simulink model "svpwm3level"  (Simulink 7.1)
settings: Solver=ode3  StartTime=0.0  StopTime=1  RelTol=1e-3
libraries: powerlib x13, simulink x1
(part 1 of 2)
settings Model: Creator=ki  LastModifiedBy=Leavy

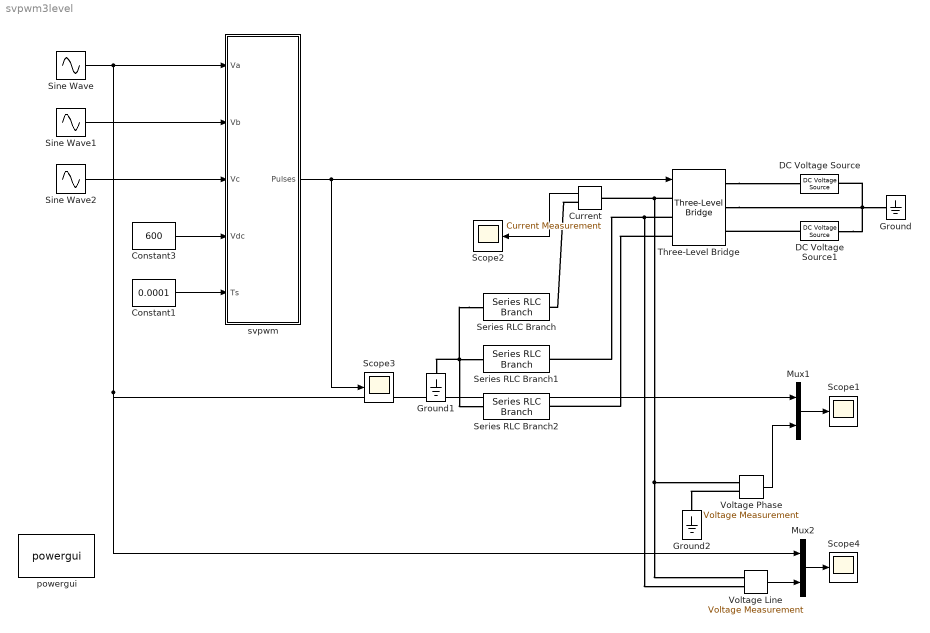
== system svpwm3level ==
  Constant1 : Constant  Value=0.0001  OutDataType=sfix(16)  OutScaling=2^0
  Constant3 : Constant  Value=600  OutDataType=sfix(16)  OutScaling=2^0
  "Current " : powerlib/Measurements/Current Measurement  Orientation=left  DialogController=POWERSYS.PowerSysDialog  SystemSampleTime=-1  PhasorSimulation=off  OutputType=Complex  PSBequivalent=0
  DC Voltage Source : powerlib/Electrical Sources/DC Voltage Source  Orientation=left  DialogController=POWERSYS.PowerSysDialog  SystemSampleTime=-1  Amplitude=300  Measurements=None
  DC Voltage Source1 : powerlib/Electrical Sources/DC Voltage Source  DialogController=POWERSYS.PowerSysDialog  SystemSampleTime=-1  Amplitude=300  Measurements=None
  Ground : powerlib/Elements/Ground  DialogController=POWERSYS.PowerSysDialog  PhysicalDomain=powersysdomain  SubClassName=unknown  LeftPortType=p1  RightPortType=p1  LConnTagsString=a
  Ground1 : powerlib/Elements/Ground  Orientation=down  DialogController=POWERSYS.PowerSysDialog  PhysicalDomain=powersysdomain  SubClassName=unknown  LeftPortType=p1  RightPortType=p1  LConnTagsString=a
  Ground2 : powerlib/Elements/Ground  Orientation=down  DialogController=POWERSYS.PowerSysDialog  PhysicalDomain=powersysdomain  SubClassName=unknown  LeftPortType=p1  RightPortType=p1  LConnTagsString=a
  Mux1 : Mux  Inputs=2
  Mux2 : Mux  Inputs=2
  Scope{1..4} (4 alike) : Scope
      Scope1 settings: TimeRange=0.01703035274815434  YMin=-350  YMax=350  MaxDataPoints=20000
      Scope2 settings: TimeRange=0.01703035274815434  YMin=-800  YMax=1500  SaveName=ScopeData2  MaxDataPoints=20000
      Scope3 settings: TimeRange=0.01703035274815434  YMin=-150  YMax=80  SaveName=ScopeData4  MaxDataPoints=20000
      Scope4 settings: TimeRange=0.01703035274815434  YMin=-700  YMax=700  SaveName=ScopeData15  MaxDataPoints=20000
  Series RLC Branch : powerlib/Elements/Series RLC Branch  DialogController=POWERSYS.PowerSysDialog  PhysicalDomain=powersysdomain  SubClassName=unknown  LeftPortType=p1  RightPortType=p1  LConnTagsString=__new0  RConnTagsString=__new0  BranchType=L  Resistance=10  Inductance=5e-4  SetiL0=off  InitialCurrent=0  Capacitance=1.0  Setx0=off  InitialVoltage=0  Measurements=None
  Series RLC Branch1 : powerlib/Elements/Series RLC Branch  DialogController=POWERSYS.PowerSysDialog  PhysicalDomain=powersysdomain  SubClassName=unknown  LeftPortType=p1  RightPortType=p1  LConnTagsString=__new0  RConnTagsString=__new0  BranchType=L  Resistance=10  Inductance=5e-4  SetiL0=off  InitialCurrent=0  Capacitance=1e-6  Setx0=off  InitialVoltage=0  Measurements=None
  Series RLC Branch2 : powerlib/Elements/Series RLC Branch  DialogController=POWERSYS.PowerSysDialog  PhysicalDomain=powersysdomain  SubClassName=unknown  LeftPortType=p1  RightPortType=p1  LConnTagsString=__new0  RConnTagsString=__new0  BranchType=L  Resistance=10  Inductance=5e-4  SetiL0=off  InitialCurrent=0  Capacitance=1e-6  Setx0=off  InitialVoltage=0  Measurements=None
  Sine Wave : Sin  Amplitude=220  Frequency=314  SampleTime=0
  Sine Wave1 : Sin  Amplitude=220  Frequency=314  Phase=-2*pi/3  SampleTime=0
  Sine Wave2 : Sin  Amplitude=220  Frequency=314  Phase=-4*pi/3  SampleTime=0
  Three-Level Bridge : powerlib/Power Electronics/Three-Level Bridge  DialogController=POWERSYS.PowerSysDialog  SystemSampleTime=-1  Arms=3  SnubberResistance=1e5  SbubberCapacitance=inf  Device=IGBT / Diodes  Ron=1e-3  ForwardVoltages="[  0  0  ]"  Measurements=None
  Voltage Line : powerlib/Measurements/Voltage Measurement  DialogController=POWERSYS.PowerSysDialog  SystemSampleTime=-1  PhasorSimulation=off  OutputType=Complex  PSBequivalent=0
  Voltage Phase : powerlib/Measurements/Voltage Measurement  DialogController=POWERSYS.PowerSysDialog  SystemSampleTime=-1  PhasorSimulation=off  OutputType=Complex  PSBequivalent=0
  powergui : powerlib/powergui  Priority=2  SystemSampleTime=-1  SimulationMode=Discrete  SampleTime=0.000002  frequency=60  SPID=off  SwTol=0  Interpol=off  x0status=blocks  echomessages=off  HookPort=off  FunctionMessages=off  EnableUseOfTLC=off  RestoreLinks=warning  frequencyindice=0  Frange=[0:2:500]  Ylog=off  Xlog=on  ShowGrid=off  save=off  variable=ZData  ZoomFFT=on  StartTime=0.0  cycles=1  DisplayStyle=1  fundamental=60  FreqAxis=off  MaxFrequency=1000  frequencyindicesteady=1  RmsSteady=1  display=off  Ts=0  methode=off
  svpwm : Subsystem
  wires:
  Constant3/1 -> svpwm/4(Vdc)
  Constant1/1 -> svpwm/5(Ts)
  svpwm/1(Pulses) -> Three-Level Bridge/1, Scope3/1
  Sine Wave2/1 -> svpwm/3(Vc)
  Sine Wave1/1 -> svpwm/2(Vb)
  Sine Wave/1 -> svpwm/1(Va), Mux1/1, Mux2/1
  "Current "/1 -> Scope2/1
  Voltage Phase/1 -> Mux1/2
  Mux1/1 -> Scope1/1
  Mux2/1 -> Scope4/1
  Voltage Line/1 -> Mux2/2
  connections:
  Three-Level Bridge/RConn1 -- DC Voltage Source/RConn1
  DC Voltage Source1/RConn1 -- DC Voltage Source/LConn1 -- Three-Level Bridge/RConn2 -- Ground/LConn1
  DC Voltage Source1/LConn1 -- Three-Level Bridge/RConn3
  Series RLC Branch/LConn1 -- Series RLC Branch1/LConn1 -- Series RLC Branch2/LConn1 -- Ground1/LConn1
  Three-Level Bridge/LConn2 -- Series RLC Branch1/RConn1 -- Voltage Line/LConn2
  Three-Level Bridge/LConn3 -- Series RLC Branch2/RConn1
  Three-Level Bridge/LConn1 -- "Current "/LConn1 -- Voltage Phase/LConn1 -- Voltage Line/LConn1
  "Current "/RConn1 -- Series RLC Branch/RConn1
  Voltage Phase/LConn2 -- Ground2/LConn1

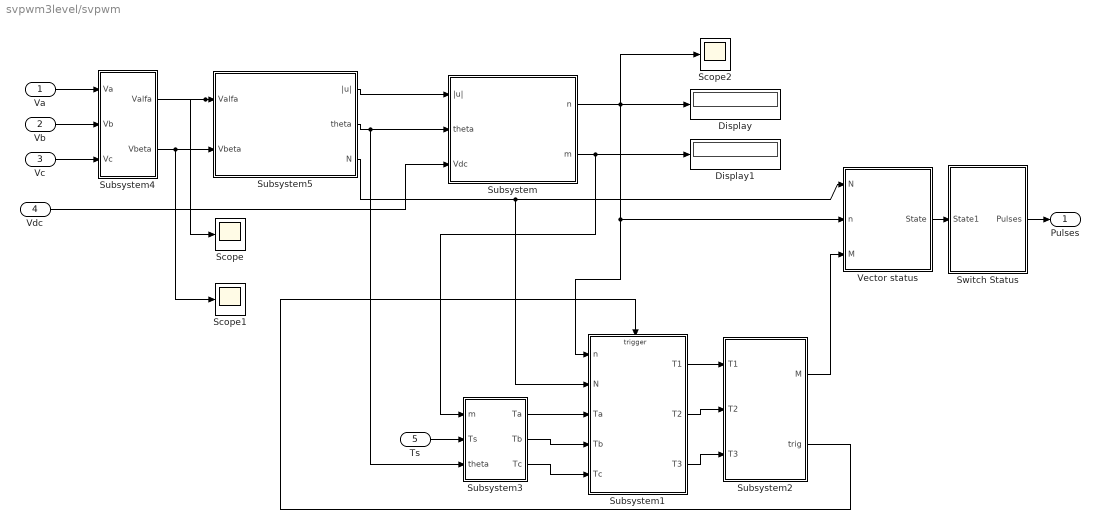
== system svpwm3level/svpwm ==
  Va : Inport  OutDataType=sfix(16)  OutScaling=2^0
  Vb : Inport  Port=2  OutDataType=sfix(16)  OutScaling=2^0
  Vc : Inport  Port=3  OutDataType=sfix(16)  OutScaling=2^0
  Vdc : Inport  Port=4  OutDataType=sfix(16)  OutScaling=2^0
  Ts : Inport  Port=5  OutDataType=sfix(16)  OutScaling=2^0
  Display : Display
  Display1 : Display
  Scope : Scope
      settings: YMin=-150  YMax=-150  SaveName=ScopeData6
  Scope1 : Scope
      settings: YMin=-606.218  YMax=-606.218  SaveName=ScopeData7
  Scope2 : Scope
      settings: YMin=3  YMax=6  SaveName=ScopeData8  MaxDataPoints=20000
  Subsystem : Subsystem
  Subsystem1 : Subsystem
  Subsystem2 : Subsystem
  Subsystem3 : Subsystem
  Subsystem4 : Subsystem
  Subsystem5 : Subsystem
  Switch Status : Subsystem
  Vector status : Subsystem
  Pulses : Outport  OutDataType=sfix(16)  OutScaling=2^0
  wires:
  Vc/1 -> Subsystem4/3(Vc)
  Subsystem4/2(Vbeta) -> Scope1/1, Subsystem5/2(Vbeta)
  Subsystem4/1(Valfa) -> Subsystem5/1(Valfa), Scope/1
  Vb/1 -> Subsystem4/2(Vb)
  Va/1 -> Subsystem4/1(Va)
  Vdc/1 -> Subsystem/3(Vdc)
  Ts/1 -> Subsystem3/2(Ts)
  Subsystem2/1(M) -> Vector status/3(M)
  Subsystem/2(m) -> Subsystem3/1(m), Display1/1
  Subsystem/1(n) -> Display/1, Scope2/1, Vector status/2(n), Subsystem1/1(n)
  Subsystem5/3(N) -> Vector status/1(N), Subsystem1/2(N)
  Subsystem5/1(|u|) -> Subsystem/1(|u|)
  Switch Status/1(Pulses) -> Pulses/1
  Vector status/1(State) -> Switch Status/1(State1)
  Subsystem5/2(theta) -> Subsystem/2(theta), Subsystem3/3(theta)
  Subsystem2/2(trig) -> Subsystem1/Trigger
  Subsystem3/1(Ta) -> Subsystem1/3(Ta)
  Subsystem3/2(Tb) -> Subsystem1/4(Tb)
  Subsystem3/3(Tc) -> Subsystem1/5(Tc)
  Subsystem1/1(T1) -> Subsystem2/1(T1)
  Subsystem1/2(T2) -> Subsystem2/2(T2)
  Subsystem1/3(T3) -> Subsystem2/3(T3)

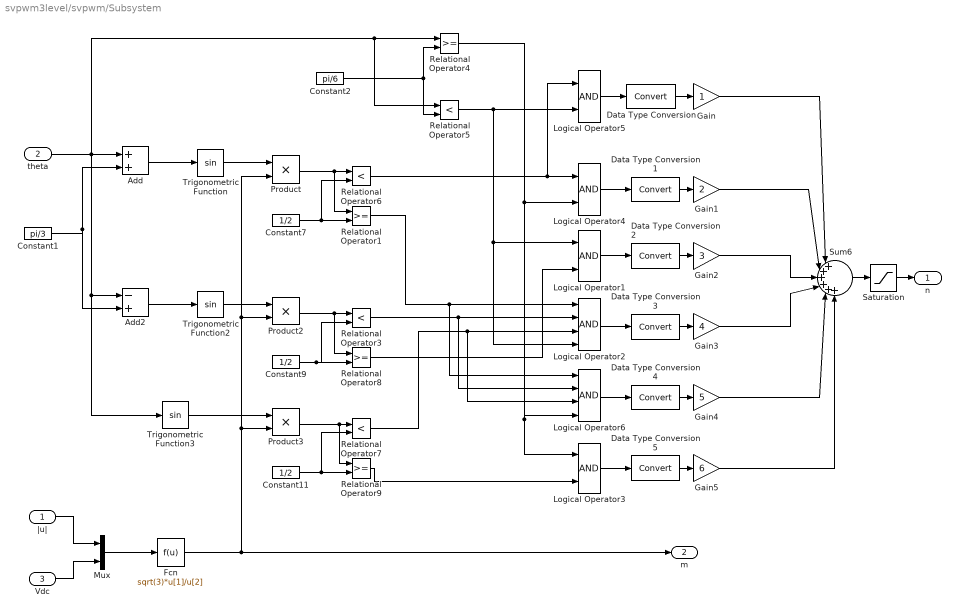
== system svpwm3level/svpwm/Subsystem ==
  |u| : Inport  OutDataType=sfix(16)  OutScaling=2^0
  theta : Inport  Port=2  OutDataType=sfix(16)  OutScaling=2^0
  Vdc : Inport  Port=3  OutDataType=sfix(16)  OutScaling=2^0
  Add : Sum  OutDataType=fixdt(1, 16)  OutScaling=2^-10
  Add2 : Sum  Inputs=-+  OutDataType=fixdt(1, 16)  OutScaling=2^-10
  Constant1 : Constant  Value=pi/3  OutDataType=sfix(16)  OutScaling=2^0
  Constant11 : Constant  Value=1/2  OutDataType=sfix(16)  OutScaling=2^0
  Constant2 : Constant  Value=pi/6  OutDataType=sfix(16)  OutScaling=2^0
  Constant7 : Constant  Value=1/2  OutDataType=sfix(16)  OutScaling=2^0
  Constant9 : Constant  Value=1/2  OutDataType=sfix(16)  OutScaling=2^0
  Data Type Conversion{,1..5} (6 alike) : DataTypeConversion  OutDataType=sfix(16)  OutScaling=2^0  SaturateOnIntegerOverflow=on  RndMeth=Zero
  Fcn : Fcn  Expr=sqrt(3)*u[1]/u[2]
  Gain : Gain  ParameterDataType=sfix(16)  ParameterScaling=2^0  OutDataType=sfix(16)  OutScaling=2^0  SaturateOnIntegerOverflow=on  OutDataTypeStr=Inherit: Same as input  ParamDataTypeStr=Inherit: Same as input
  Gain1 : Gain  Gain=2  ParameterDataType=sfix(16)  ParameterScaling=2^0  OutDataType=sfix(16)  OutScaling=2^0  SaturateOnIntegerOverflow=on  OutDataTypeStr=Inherit: Same as input  ParamDataTypeStr=Inherit: Same as input
  Gain2 : Gain  Gain=3  ParameterDataType=sfix(16)  ParameterScaling=2^0  OutDataType=sfix(16)  OutScaling=2^0  SaturateOnIntegerOverflow=on  OutDataTypeStr=Inherit: Same as input  ParamDataTypeStr=Inherit: Same as input
  Gain3 : Gain  Gain=4  ParameterDataType=sfix(16)  ParameterScaling=2^0  OutDataType=sfix(16)  OutScaling=2^0  SaturateOnIntegerOverflow=on  OutDataTypeStr=Inherit: Same as input  ParamDataTypeStr=Inherit: Same as input
  Gain4 : Gain  Gain=5  ParameterDataType=sfix(16)  ParameterScaling=2^0  OutDataType=sfix(16)  OutScaling=2^0  SaturateOnIntegerOverflow=on  OutDataTypeStr=Inherit: Same as input  ParamDataTypeStr=Inherit: Same as input
  Gain5 : Gain  Gain=6  ParameterDataType=sfix(16)  ParameterScaling=2^0  OutDataType=sfix(16)  OutScaling=2^0  SaturateOnIntegerOverflow=on  OutDataTypeStr=Inherit: Same as input  ParamDataTypeStr=Inherit: Same as input
  Logical Operator{1,3..5} (4 alike) : Logic
  Logical Operator2 : Logic  Inputs=4
  Logical Operator6 : Logic  Inputs=4
  Mux : Mux  Inputs=2
  Product : Product  OutDataType=fixdt(1, 16)  OutScaling=2^0  RndMeth=Zero
  Product2 : Product  OutDataType=fixdt(1, 16)  OutScaling=2^0  RndMeth=Zero
  Product3 : Product  OutDataType=fixdt(1, 16)  OutScaling=2^0  RndMeth=Zero
  Relational Operator{1,4,8..9} (4 alike) : RelationalOperator  InputSameDT=on
  Relational Operator{3,5..7} (4 alike) : RelationalOperator  Operator=<  InputSameDT=on
  Saturation : Saturate  UpperLimit=6  LowerLimit=1
  Sum6 : Sum  Inputs=|++++++  OutDataType=sfix(16)  OutScaling=2^0  InputSameDT=on  OutDataTypeStr=Inherit: Same as first input
  Trigonometric Function : Trigonometry
  Trigonometric Function2 : Trigonometry
  Trigonometric Function3 : Trigonometry
  n : Outport  OutDataType=sfix(16)  OutScaling=2^0
  m : Outport  Port=2  OutDataType=sfix(16)  OutScaling=2^0
  wires:
  Mux/1 -> Fcn/1
  Fcn/1 -> Product3/2, Product2/2, Product/2, m/1
  |u|/1 -> Mux/1
  Vdc/1 -> Mux/2
  Trigonometric Function/1 -> Product/1
  Product/1 -> Relational Operator6/1, Relational Operator1/1
  Constant7/1 -> Relational Operator6/2, Relational Operator1/2
  Trigonometric Function2/1 -> Product2/1
  Product2/1 -> Relational Operator3/1, Relational Operator8/1
  Constant9/1 -> Relational Operator3/2, Relational Operator8/2
  Trigonometric Function3/1 -> Product3/1
  Product3/1 -> Relational Operator7/1, Relational Operator9/1
  Constant11/1 -> Relational Operator7/2, Relational Operator9/2
  Constant2/1 -> Relational Operator4/2, Relational Operator5/2
  Relational Operator1/1 -> Logical Operator2/1, Logical Operator6/1
  Relational Operator3/1 -> Logical Operator2/2, Logical Operator6/2
  Relational Operator7/1 -> Logical Operator2/3, Logical Operator6/3
  Relational Operator9/1 -> Logical Operator3/2
  Relational Operator8/1 -> Logical Operator1/2
  Relational Operator4/1 -> Logical Operator4/2, Logical Operator3/1, Logical Operator6/4
  Relational Operator5/1 -> Logical Operator5/2, Logical Operator1/1, Logical Operator2/4
  Add/1 -> Trigonometric Function/1
  Relational Operator6/1 -> Logical Operator4/1, Logical Operator5/1
  theta/1 -> Add/1, Add2/1, Trigonometric Function3/1, Relational Operator4/1, Relational Operator5/1
  Constant1/1 -> Add/2, Add2/2
  Add2/1 -> Trigonometric Function2/1
  Data Type Conversion/1 -> Gain/1
  Data Type Conversion1/1 -> Gain1/1
  Data Type Conversion2/1 -> Gain2/1
  Data Type Conversion3/1 -> Gain3/1
  Data Type Conversion4/1 -> Gain4/1
  Data Type Conversion5/1 -> Gain5/1
  Logical Operator3/1 -> Data Type Conversion5/1
  Logical Operator6/1 -> Data Type Conversion4/1
  Logical Operator2/1 -> Data Type Conversion3/1
  Logical Operator1/1 -> Data Type Conversion2/1
  Logical Operator5/1 -> Data Type Conversion/1
  Logical Operator4/1 -> Data Type Conversion1/1
  Sum6/1 -> Saturation/1
  Saturation/1 -> n/1
  Gain/1 -> Sum6/1
  Gain1/1 -> Sum6/2
  Gain2/1 -> Sum6/3
  Gain3/1 -> Sum6/4
  Gain4/1 -> Sum6/5
  Gain5/1 -> Sum6/6

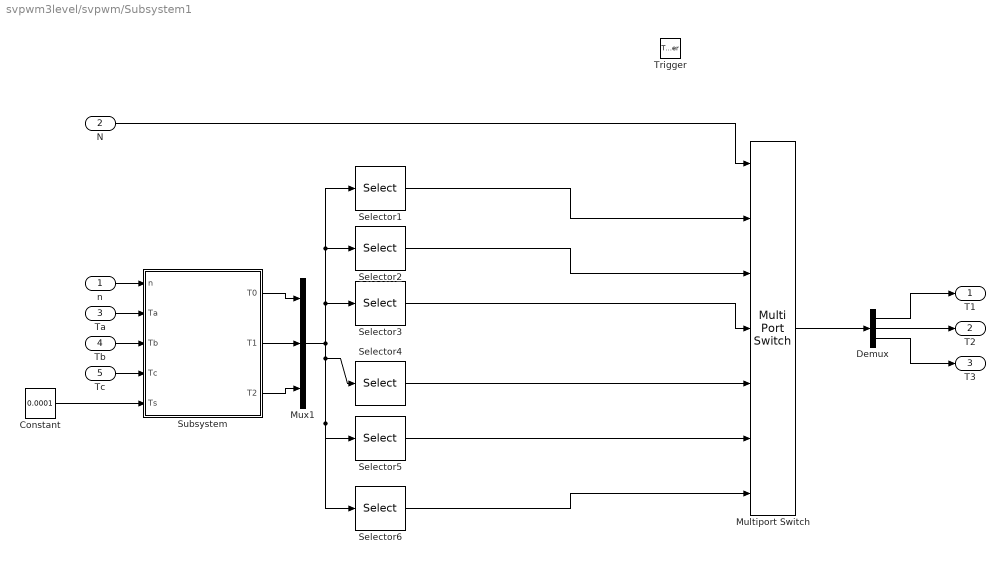
== system svpwm3level/svpwm/Subsystem1 ==
  n : Inport  OutDataType=sfix(16)  OutScaling=2^0
  N : Inport  Port=2  OutDataType=sfix(16)  OutScaling=2^0
  Ta : Inport  Port=3  OutDataType=sfix(16)  OutScaling=2^0
  Tb : Inport  Port=4  OutDataType=sfix(16)  OutScaling=2^0
  Tc : Inport  Port=5  OutDataType=sfix(16)  OutScaling=2^0
  Trigger : TriggerPort
  Constant : Constant  Value=0.0001  OutDataType=fixdt(1, 16)  OutScaling=2^0
  Demux : Demux  Outputs=3
  Multiport Switch : MultiPortSwitch  Inputs=6  OutDataType=sfix(16)  OutScaling=2^0  InputSameDT=on
  Mux1 : Mux  Inputs=3
  Selector1 : Selector  InputPortWidth=3  IndexOptions=Index vector (dialog)  Indices="[1 2  3]"  OutputSizes=1
  Selector2 : Selector  InputPortWidth=3  IndexOptions=Index vector (dialog)  Indices=[1 3 2]  OutputSizes=1
  Selector3 : Selector  InputPortWidth=3  IndexOptions=Index vector (dialog)  Indices=[1 2 3]  OutputSizes=1
  Selector4 : Selector  InputPortWidth=3  IndexOptions=Index vector (dialog)  Indices=[1 3 2]  OutputSizes=1
  Selector5 : Selector  InputPortWidth=3  IndexOptions=Index vector (dialog)  Indices="[1 2  3]"  OutputSizes=1
  Selector6 : Selector  InputPortWidth=3  IndexOptions=Index vector (dialog)  Indices=[ 1 3 2]  OutputSizes=1
  Subsystem : Subsystem
  T1 : Outport  OutDataType=sfix(16)  OutScaling=2^0
  T2 : Outport  Port=2  OutDataType=sfix(16)  OutScaling=2^0
  T3 : Outport  Port=3  OutDataType=sfix(16)  OutScaling=2^0
  wires:
  Ta/1 -> Subsystem/2(Ta)
  Tb/1 -> Subsystem/3(Tb)
  Tc/1 -> Subsystem/4(Tc)
  n/1 -> Subsystem/1(n)
  Constant/1 -> Subsystem/5(Ts)
  N/1 -> Multiport Switch/1
  Multiport Switch/1 -> Demux/1
  Demux/1 -> T1/1
  Demux/2 -> T2/1
  Demux/3 -> T3/1
  Subsystem/1(T0) -> Mux1/1
  Subsystem/2(T1) -> Mux1/2
  Subsystem/3(T2) -> Mux1/3
  Mux1/1 -> Selector1/1, Selector2/1, Selector3/1, Selector4/1, Selector5/1, Selector6/1
  Selector1/1 -> Multiport Switch/2
  Selector2/1 -> Multiport Switch/3
  Selector3/1 -> Multiport Switch/4
  Selector4/1 -> Multiport Switch/5
  Selector5/1 -> Multiport Switch/6
  Selector6/1 -> Multiport Switch/7

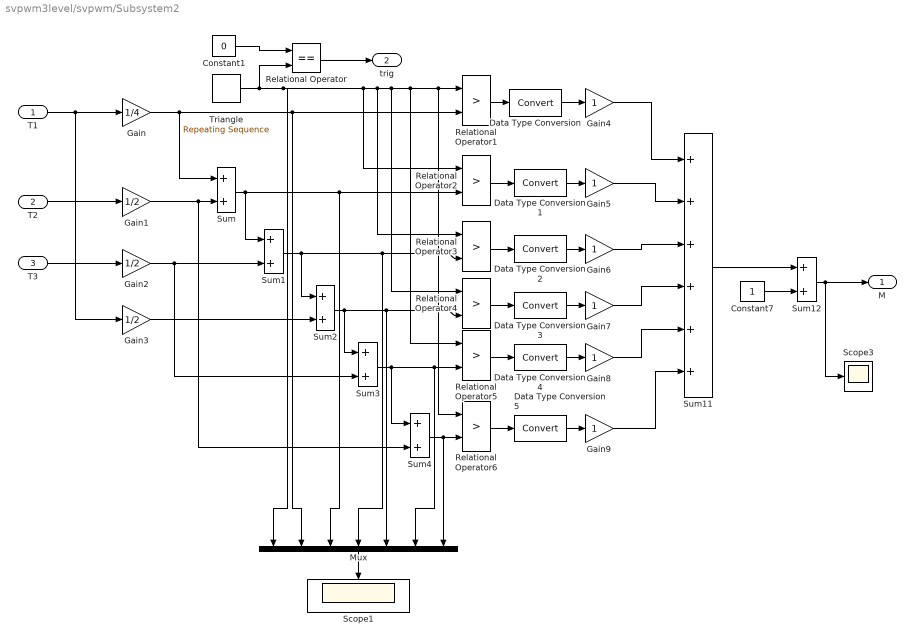
== system svpwm3level/svpwm/Subsystem2 ==
  T1 : Inport  OutDataType=sfix(16)  OutScaling=2^0
  T2 : Inport  Port=2  OutDataType=sfix(16)  OutScaling=2^0
  T3 : Inport  Port=3  OutDataType=sfix(16)  OutScaling=2^0
  Constant1 : Constant  Value=0  OutDataType=sfix(16)  OutScaling=2^0
  Constant7 : Constant  OutDataType=sfix(16)  OutScaling=2^0
  Data Type Conversion{,1..5} (6 alike) : DataTypeConversion  OutDataType=sfix(16)  OutScaling=2^0  SaturateOnIntegerOverflow=on  RndMeth=Zero
  Gain : Gain  Gain=1/4  ParameterDataType=sfix(16)  ParameterScaling=2^0  OutDataType=sfix(16)  OutScaling=2^0
  Gain1 : Gain  Gain=1/2  ParameterDataType=sfix(16)  ParameterScaling=2^0  OutDataType=sfix(16)  OutScaling=2^0
  Gain2 : Gain  Gain=1/2  ParameterDataType=sfix(16)  ParameterScaling=2^0  OutDataType=sfix(16)  OutScaling=2^0
  Gain3 : Gain  Gain=1/2  ParameterDataType=sfix(16)  ParameterScaling=2^0  OutDataType=sfix(16)  OutScaling=2^0
  Gain{4..9} (6 alike) : Gain  ParameterDataType=sfix(16)  ParameterScaling=2^0  OutDataType=sfix(16)  OutScaling=2^0  SaturateOnIntegerOverflow=on  OutDataTypeStr=Inherit: Same as input  ParamDataTypeStr=Inherit: Same as input
  Mux : Mux  Orientation=down  Inputs=7
  Relational Operator : RelationalOperator  Operator===  LogicOutDataTypeMode=boolean  LogicDataType=fixdt(0, 8)  OutDataTypeStr=boolean
  Relational Operator{1..6} (6 alike) : RelationalOperator  Operator=>  LogicOutDataTypeMode=boolean  LogicDataType=fixdt(0, 8)  OutDataTypeStr=boolean
  Scope1 : Scope
      settings: Orientation=down  TimeRange=0.01400000000000001  YMin=0  YMax=0.0001  SaveName=ScopeData24  MaxDataPoints=20000
  Scope3 : Scope
      settings: TimeRange=10  YMin=1  YMax=7  MaxDataPoints=20000
  Sum{,1..4,12} (6 alike) : Sum  OutDataType=sfix(16)  OutScaling=2^0  SaturateOnIntegerOverflow=on
  Sum11 : Sum  Inputs=++++++  OutDataType=sfix(16)  OutScaling=2^0  SaturateOnIntegerOverflow=on
  Triangle : simulink/Sources/Repeating Sequence  SystemSampleTime=-1  rep_seq_t="[0  0.0001]"  rep_seq_y="[0  0.0001]"
  M : Outport  OutDataType=sfix(16)  OutScaling=2^0
  trig : Outport  Port=2  OutDataType=sfix(16)  OutScaling=2^0
  wires:
  T1/1 -> Gain/1, Gain3/1
  T2/1 -> Gain1/1
  Gain/1 -> Sum/1, Relational Operator1/2, Mux/2
  Triangle/1 -> Relational Operator/2, Relational Operator1/1, Relational Operator6/1, Relational Operator5/1, Relational Operator4/1, Relational Operator3/1, Relational Operator2/1, Mux/1
  Gain1/1 -> Sum/2, Sum4/2
  Sum/1 -> Sum1/1, Relational Operator2/2, Mux/3
  Sum1/1 -> Sum2/1, Relational Operator3/2, Mux/4
  Sum3/1 -> Sum4/1, Relational Operator5/2, Mux/6
  Sum4/1 -> Relational Operator6/2, Mux/7
  Gain4/1 -> Sum11/1
  Gain5/1 -> Sum11/2
  Gain9/1 -> Sum11/6
  Sum11/1 -> Sum12/1
  Constant7/1 -> Sum12/2
  Sum12/1 -> M/1, Scope3/1
  Constant1/1 -> Relational Operator/1
  Relational Operator/1 -> trig/1
  Gain2/1 -> Sum1/2, Sum3/2
  T3/1 -> Gain2/1
  Sum2/1 -> Sum3/1, Relational Operator4/2, Mux/5
  Gain3/1 -> Sum2/2
  Relational Operator1/1 -> Data Type Conversion/1
  Relational Operator6/1 -> Data Type Conversion5/1
  Relational Operator5/1 -> Data Type Conversion4/1
  Relational Operator4/1 -> Data Type Conversion3/1
  Relational Operator3/1 -> Data Type Conversion2/1
  Relational Operator2/1 -> Data Type Conversion1/1
  Data Type Conversion/1 -> Gain4/1
  Data Type Conversion1/1 -> Gain5/1
  Data Type Conversion5/1 -> Gain9/1
  Data Type Conversion4/1 -> Gain8/1
  Gain6/1 -> Sum11/3
  Gain7/1 -> Sum11/4
  Gain8/1 -> Sum11/5
  Data Type Conversion3/1 -> Gain7/1
  Data Type Conversion2/1 -> Gain6/1
  Mux/1 -> Scope1/1

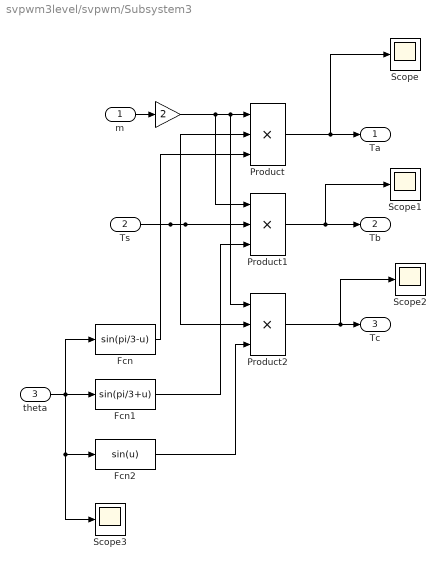
== system svpwm3level/svpwm/Subsystem3 ==
  m : Inport  OutDataType=sfix(16)  OutScaling=2^0
  Ts : Inport  Port=2  OutDataType=sfix(16)  OutScaling=2^0
  theta : Inport  Port=3  OutDataType=sfix(16)  OutScaling=2^0
  "  " : Gain  Gain=2  ParameterDataType=sfix(16)  ParameterScaling=2^0  OutDataType=sfix(16)  OutScaling=2^0  SaturateOnIntegerOverflow=on  OutDataTypeStr=Inherit: Same as input  ParamDataTypeStr=Inherit: Same as input
  Fcn : Fcn  Expr=sin(pi/3-u)
  Fcn1 : Fcn  Expr=sin(pi/3+u)
  Fcn2 : Fcn  Expr=sin(u)
  Product : Product  Inputs=3  OutDataType=sfix(16)  OutScaling=2^0  SaturateOnIntegerOverflow=on  OutDataTypeStr=Inherit: Same as first input
  Product1 : Product  Inputs=3  OutDataType=sfix(16)  OutScaling=2^0  SaturateOnIntegerOverflow=on  OutDataTypeStr=Inherit: Same as first input
  Product2 : Product  Inputs=3  OutDataType=sfix(16)  OutScaling=2^0  SaturateOnIntegerOverflow=on  OutDataTypeStr=Inherit: Same as first input
  Scope{,1..3} (4 alike) : Scope
      Scope settings: YMin=8.22724e-005  YMax=9.09326e-005  SaveName=ScopeData9
      Scope1 settings: TimeRange=0.1200000000000001  YMin=0.000164545  YMax=0.000181865  SaveName=ScopeData10
      Scope2 settings: YMin=-8.13152e-020  YMax=0.0016  SaveName=ScopeData11
      Scope3 settings: YMin=5.55112e-017  YMax=1  SaveName=ScopeData14
  Ta : Outport  OutDataType=sfix(16)  OutScaling=2^0
  Tb : Outport  Port=2  OutDataType=sfix(16)  OutScaling=2^0
  Tc : Outport  Port=3  OutDataType=sfix(16)  OutScaling=2^0
  wires:
  m/1 -> "  "/1
  Ts/1 -> Product2/2, Product1/2, Product/2
  theta/1 -> Fcn1/1, Fcn/1, Fcn2/1, Scope3/1
  Fcn2/1 -> Product2/3
  Fcn1/1 -> Product1/3
  Fcn/1 -> Product/3
  Product2/1 -> Tc/1, Scope2/1
  Product/1 -> Ta/1, Scope/1
  "  "/1 -> Product/1, Product2/1, Product1/1
  Product1/1 -> Tb/1, Scope1/1

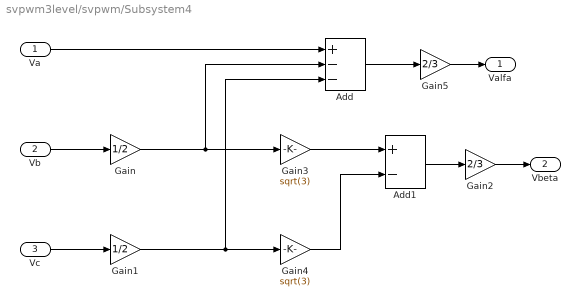
== system svpwm3level/svpwm/Subsystem4 ==
  Va : Inport  OutDataType=sfix(16)  OutScaling=2^0
  Vb : Inport  Port=2  OutDataType=sfix(16)  OutScaling=2^0
  Vc : Inport  Port=3  OutDataType=sfix(16)  OutScaling=2^0
  Add : Sum  Inputs=+--  OutDataType=fixdt(1, 16)  OutScaling=2^-10
  Add1 : Sum  Inputs=+-  OutDataType=fixdt(1, 16)  OutScaling=2^-10
  Gain : Gain  Gain=1/2  ParameterDataType=fixdt(1, 16)  ParameterScaling=2^0  OutDataType=fixdt(1, 16)  OutScaling=2^0
  Gain1 : Gain  Gain=1/2  ParameterDataType=fixdt(1, 16)  ParameterScaling=2^0  OutDataType=fixdt(1, 16)  OutScaling=2^0
  Gain2 : Gain  Gain=2/3  ParameterDataType=sfix(16)  ParameterScaling=2^0  OutDataType=sfix(16)  OutScaling=2^0
  Gain3 : Gain  Gain=sqrt(3)  ParameterDataType=fixdt(1, 16)  ParameterScaling=2^0  OutDataType=fixdt(1, 16)  OutScaling=2^0
  Gain4 : Gain  Gain=sqrt(3)  ParameterDataType=fixdt(1, 16)  ParameterScaling=2^0  OutDataType=fixdt(1, 16)  OutScaling=2^0
  Gain5 : Gain  Gain=2/3  ParameterDataType=sfix(16)  ParameterScaling=2^0  OutDataType=sfix(16)  OutScaling=2^0
  Valfa : Outport  OutDataType=sfix(16)  OutScaling=2^0
  Vbeta : Outport  Port=2  OutDataType=sfix(16)  OutScaling=2^0
  wires:
  Vc/1 -> Gain1/1
  Vb/1 -> Gain/1
  Va/1 -> Add/1
  Gain/1 -> Add/2, Gain3/1
  Gain1/1 -> Add/3, Gain4/1
  Gain3/1 -> Add1/1
  Gain4/1 -> Add1/2
  Add1/1 -> Gain2/1
  Gain2/1 -> Vbeta/1
  Gain5/1 -> Valfa/1
  Add/1 -> Gain5/1

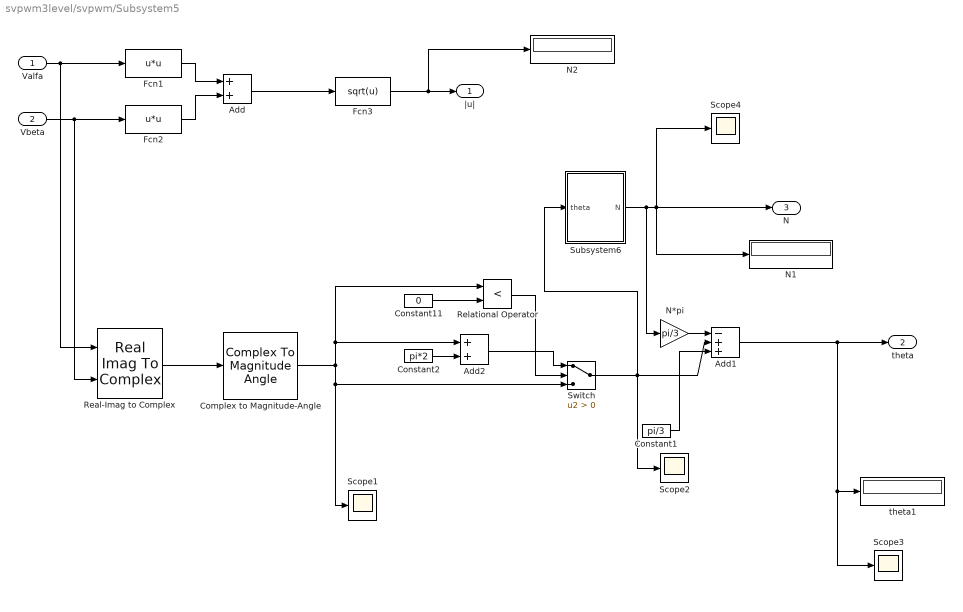
== system svpwm3level/svpwm/Subsystem5 ==
  Valfa : Inport  OutDataType=sfix(16)  OutScaling=2^0
  Vbeta : Inport  Port=2  OutDataType=sfix(16)  OutScaling=2^0
  Add : Sum  OutDataType=fixdt(1, 16)  OutScaling=2^-10
  Add1 : Sum  Inputs=-++  OutDataType=fixdt(1, 16)  OutScaling=2^-10
  Add2 : Sum  OutDataType=fixdt(1, 16)  OutScaling=2^-10
  Complex to Magnitude-Angle : ComplexToMagnitudeAngle  Output=Angle
  Constant1 : Constant  Value=pi/3  OutDataType=sfix(16)  OutScaling=2^0
  Constant11 : Constant  Value=0  OutDataType=sfix(16)  OutScaling=2^0
  Constant2 : Constant  Value=pi*2  OutDataType=sfix(16)  OutScaling=2^0
  Fcn1 : Fcn  Expr=u*u
  Fcn2 : Fcn  Expr=u*u
  Fcn3 : Fcn  Expr=sqrt(u)
  N*pi : Gain  Gain=pi/3  ParameterDataType=sfix(16)  ParameterScaling=2^0  OutDataType=sfix(16)  OutScaling=2^0  SaturateOnIntegerOverflow=on  OutDataTypeStr=Inherit: Same as input  ParamDataTypeStr=Inherit: Same as input
  N1 : Display
  N2 : Display
  Real-Imag to Complex : RealImagToComplex
  Relational Operator : RelationalOperator  Operator=<  LogicOutDataTypeMode=boolean  LogicDataType=fixdt(0, 8)  OutDataTypeStr=boolean
  Scope{1..4} (4 alike) : Scope
      Scope1 settings: TimeRange=0.12  YMin=-1.81336  YMax=-1.81336  SaveName=ScopeData5
      Scope2 settings: YMin=4.46983  YMax=4.46983  SaveName=ScopeData3
      Scope3 settings: YMin=2.77556e-017  YMax=1.05  SaveName=ScopeData22
      Scope4 settings: YMin=1.49226  YMax=1.64934  SaveName=ScopeData25  MaxDataPoints=20000
  Subsystem6 : Subsystem
  Switch : Switch  Criteria=u2 > Threshold  OutDataType=fixdt(1, 16)  OutScaling=2^0
  theta1 : Display
  |u| : Outport  OutDataType=sfix(16)  OutScaling=2^0
  theta : Outport  Port=2  OutDataType=sfix(16)  OutScaling=2^0
  N : Outport  Port=3  OutDataType=sfix(16)  OutScaling=2^0
  wires:
  Valfa/1 -> Fcn1/1, Real-Imag to Complex/1
  Vbeta/1 -> Fcn2/1, Real-Imag to Complex/2
  Fcn1/1 -> Add/1
  Fcn2/1 -> Add/2
  Add/1 -> Fcn3/1
  Fcn3/1 -> |u|/1, N2/1
  Subsystem6/1(N) -> N1/1, N/1, Scope4/1, N*pi/1
  Constant11/1 -> Relational Operator/2
  Relational Operator/1 -> Switch/2
  Switch/1 -> Add1/2, Subsystem6/1(theta), Scope2/1
  N*pi/1 -> Add1/1
  Constant1/1 -> Add1/3
  Add1/1 -> theta/1, Scope3/1, theta1/1
  Real-Imag to Complex/1 -> Complex to Magnitude-Angle/1
  Complex to Magnitude-Angle/1 -> Relational Operator/1, Add2/1, Scope1/1, Switch/3
  Constant2/1 -> Add2/2
  Add2/1 -> Switch/1

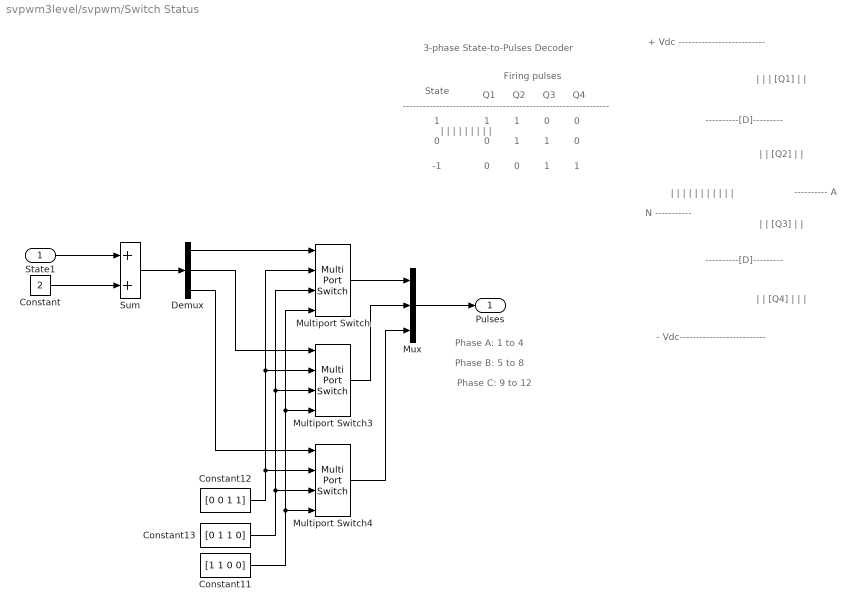
== system svpwm3level/svpwm/Switch Status ==
  note: State
  note: 1
  note: Firing pulses
  note: 1
  note: 1
  note: 0
  note: 0
  note: Q1
  note: Q2
  note: Q3
  note: Q4
  note: 0
  note: 0
  note: 1
  note: 1
  note: 0
  note: -1
  note: 0
  note: 0
  note: 1
  note: 1
  note: |
      | |
      | |
      | |
      | |
      | |
      | |
      | |
      | |
  note: --------------------------------------------------------------
  note: 3-phase State-to-Pulses Decoder
  note: Phase B: 5 to 8
  note: Phase A: 1 to 4
  note: Phase C: 9 to 12
  note: |
      | |
      | |
      | [Q1]
      | |
      | |
  note: |
      | |
      | [Q2]
      | |
      | |
  note: |
      | |
      | [Q3]
      | |
      | |
  note: |
      | |
      | [Q4]
      | |
      | |
      | |
  note: ----------[D]---------
  note: ----------[D]---------
  note: ---------- A
  note: |
      | |
      | |
      | |
      | |
      | |
      | |
      | |
      | |
      | |
      | |
  note: N -----------
  note: - Vdc--------------------------
  note: + Vdc --------------------------
  State1 : Inport  PortDimensions=3  OutDataType=sfix(16)  OutScaling=2^0
  Constant : Constant  Value=2  OutDataType=sfix(16)  OutScaling=2^0
  Constant11 : Constant  Value=[1 1 0 0]  OutDataType=sfix(16)  OutScaling=2^0
  Constant12 : Constant  Value=[0 0 1 1]  OutDataType=sfix(16)  OutScaling=2^0
  Constant13 : Constant  Value=[0 1 1 0]  OutDataType=sfix(16)  OutScaling=2^0
  Demux : Demux  Outputs=3
  Multiport Switch : MultiPortSwitch  OutDataType=sfix(16)  OutScaling=2^0  InputSameDT=on
  Multiport Switch3 : MultiPortSwitch  OutDataType=sfix(16)  OutScaling=2^0  InputSameDT=on
  Multiport Switch4 : MultiPortSwitch  OutDataType=sfix(16)  OutScaling=2^0  InputSameDT=on
  Mux : Mux  Inputs=[4 4 4]
  Sum : Sum  OutDataType=sfix(16)  OutScaling=2^0  SaturateOnIntegerOverflow=on  InputSameDT=on  OutDataTypeStr=Inherit: Same as first input
  Pulses : Outport  OutDataType=sfix(16)  OutScaling=2^0
  wires:
  Mux/1 -> Pulses/1
  Sum/1 -> Demux/1
  Demux/1 -> Multiport Switch/1
  Demux/2 -> Multiport Switch3/1
  Demux/3 -> Multiport Switch4/1
  Constant12/1 -> Multiport Switch/2, Multiport Switch3/2, Multiport Switch4/2
  Constant13/1 -> Multiport Switch/3, Multiport Switch3/3, Multiport Switch4/3
  Constant11/1 -> Multiport Switch/4, Multiport Switch3/4, Multiport Switch4/4
  Multiport Switch/1 -> Mux/1
  Multiport Switch3/1 -> Mux/2
  Multiport Switch4/1 -> Mux/3
  State1/1 -> Sum/1
  Constant/1 -> Sum/2

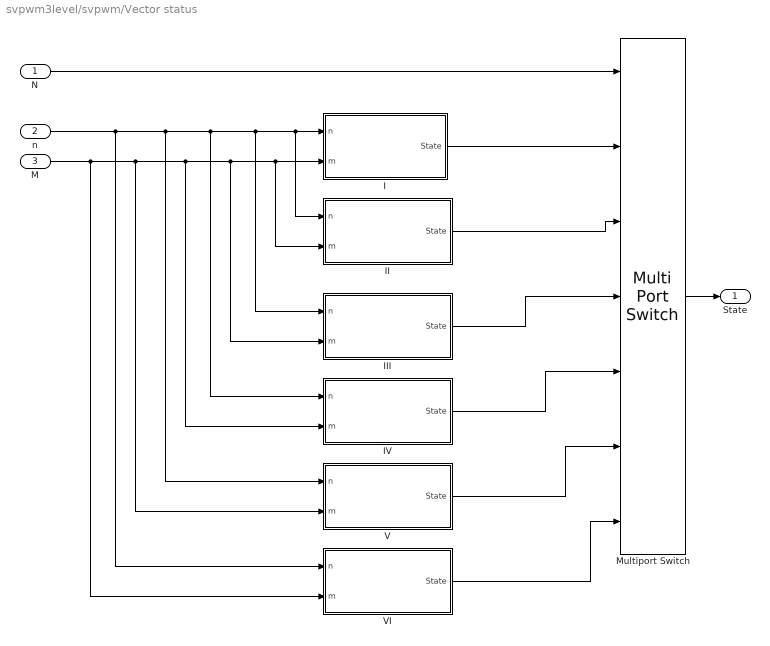
== system svpwm3level/svpwm/Vector status ==
  N : Inport  OutDataType=sfix(16)  OutScaling=2^0
  n : Inport  Port=2  OutDataType=sfix(16)  OutScaling=2^0
  M : Inport  Port=3  OutDataType=sfix(16)  OutScaling=2^0
  I : Subsystem
  II : Subsystem
  III : Subsystem
  IV : Subsystem
  Multiport Switch : MultiPortSwitch  Inputs=6  OutDataType=sfix(16)  OutScaling=2^0  InputSameDT=on
  V : Subsystem
  VI : Subsystem
  State : Outport  OutDataType=sfix(16)  OutScaling=2^0
  wires:
  II/1(State) -> Multiport Switch/3
  n/1 -> I/1(n), II/1(n), III/1(n), IV/1(n), V/1(n), VI/1(n)
  M/1 -> I/2(m), II/2(m), III/2(m), IV/2(m), V/2(m), VI/2(m)
  I/1(State) -> Multiport Switch/2
  III/1(State) -> Multiport Switch/4
  IV/1(State) -> Multiport Switch/5
  V/1(State) -> Multiport Switch/6
  VI/1(State) -> Multiport Switch/7
  Multiport Switch/1 -> State/1
  N/1 -> Multiport Switch/1

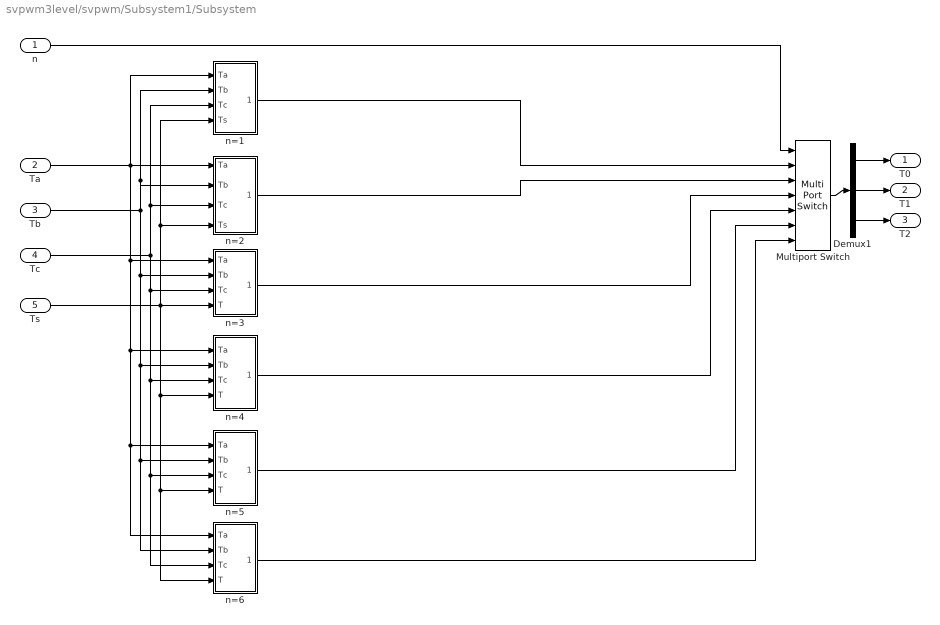
== system svpwm3level/svpwm/Subsystem1/Subsystem ==
  n : Inport  OutDataType=sfix(16)  OutScaling=2^0
  Ta : Inport  Port=2  OutDataType=sfix(16)  OutScaling=2^0
  Tb : Inport  Port=3  OutDataType=sfix(16)  OutScaling=2^0
  Tc : Inport  Port=4  OutDataType=sfix(16)  OutScaling=2^0
  Ts : Inport  Port=5  OutDataType=sfix(16)  OutScaling=2^0
  Demux1 : Demux  Outputs=3
  Multiport Switch : MultiPortSwitch  Inputs=6  OutDataType=sfix(16)  OutScaling=2^0  InputSameDT=on
  n=1 : Subsystem
  n=2 : Subsystem
  n=3 : Subsystem
  n=4 : Subsystem
  n=5 : Subsystem
  n=6 : Subsystem
  T0 : Outport  OutDataType=sfix(16)  OutScaling=2^0
  T1 : Outport  Port=2  OutDataType=sfix(16)  OutScaling=2^0
  T2 : Outport  Port=3  OutDataType=sfix(16)  OutScaling=2^0
  wires:
  Ta/1 -> n=1/1(Ta), n=3/1(Ta), n=4/1(Ta), n=5/1(Ta), n=6/1(Ta), n=2/1(Ta)
  n/1 -> Multiport Switch/1
  Multiport Switch/1 -> Demux1/1
  Demux1/1 -> T0/1
  Demux1/2 -> T1/1
  Demux1/3 -> T2/1
  n=1/1(Tout) -> Multiport Switch/2
  n=2/1(Tout) -> Multiport Switch/3
  n=3/1(Tout) -> Multiport Switch/4
  n=4/1(Tout) -> Multiport Switch/5
  n=5/1(Tout) -> Multiport Switch/6
  n=6/1(Tout) -> Multiport Switch/7
  Ts/1 -> n=2/4(Ts), n=1/4(Ts), n=4/4(T), n=6/4(T), n=5/4(T), n=3/4(T)
  Tb/1 -> n=1/2(Tb), n=2/2(Tb), n=3/2(Tb), n=4/2(Tb), n=5/2(Tb), n=6/2(Tb)
  Tc/1 -> n=1/3(Tc), n=2/3(Tc), n=3/3(Tc), n=4/3(Tc), n=5/3(Tc), n=6/3(Tc)

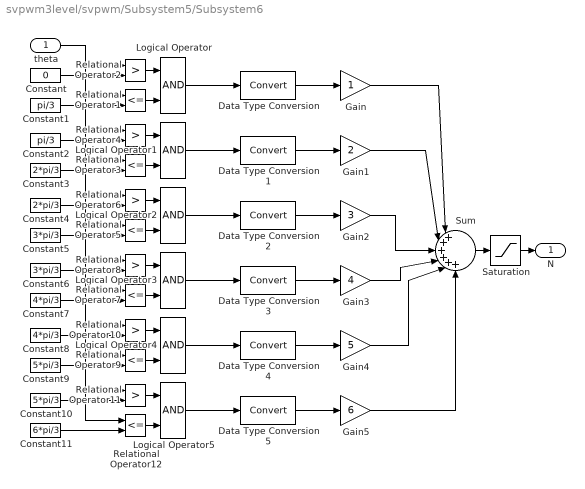
== system svpwm3level/svpwm/Subsystem5/Subsystem6 ==
  theta : Inport  OutDataType=sfix(16)  OutScaling=2^0
  Constant : Constant  Value=0  OutDataType=sfix(16)  OutScaling=2^0
  Constant1 : Constant  Value=pi/3  OutDataType=sfix(16)  OutScaling=2^0
  Constant10 : Constant  Value=5*pi/3  OutDataType=sfix(16)  OutScaling=2^0
  Constant11 : Constant  Value=6*pi/3  OutDataType=sfix(16)  OutScaling=2^0
  Constant2 : Constant  Value=pi/3  OutDataType=sfix(16)  OutScaling=2^0
  Constant3 : Constant  Value=2*pi/3  OutDataType=sfix(16)  OutScaling=2^0
  Constant4 : Constant  Value=2*pi/3  OutDataType=sfix(16)  OutScaling=2^0
  Constant5 : Constant  Value=3*pi/3  OutDataType=sfix(16)  OutScaling=2^0
  Constant6 : Constant  Value=3*pi/3  OutDataType=sfix(16)  OutScaling=2^0
  Constant7 : Constant  Value=4*pi/3  OutDataType=sfix(16)  OutScaling=2^0
  Constant8 : Constant  Value=4*pi/3  OutDataType=sfix(16)  OutScaling=2^0
  Constant9 : Constant  Value=5*pi/3  OutDataType=sfix(16)  OutScaling=2^0
  Data Type Conversion{,1..5} (6 alike) : DataTypeConversion  OutDataType=sfix(16)  OutScaling=2^0  SaturateOnIntegerOverflow=on  RndMeth=Zero
  Gain : Gain  ParameterDataType=sfix(16)  ParameterScaling=2^0  OutDataType=sfix(16)  OutScaling=2^0  SaturateOnIntegerOverflow=on  OutDataTypeStr=Inherit: Same as input  ParamDataTypeStr=Inherit: Same as input
  Gain1 : Gain  Gain=2  ParameterDataType=sfix(16)  ParameterScaling=2^0  OutDataType=sfix(16)  OutScaling=2^0  SaturateOnIntegerOverflow=on  OutDataTypeStr=Inherit: Same as input  ParamDataTypeStr=Inherit: Same as input
  Gain2 : Gain  Gain=3  ParameterDataType=sfix(16)  ParameterScaling=2^0  OutDataType=sfix(16)  OutScaling=2^0  SaturateOnIntegerOverflow=on  OutDataTypeStr=Inherit: Same as input  ParamDataTypeStr=Inherit: Same as input
  Gain3 : Gain  Gain=4  ParameterDataType=sfix(16)  ParameterScaling=2^0  OutDataType=sfix(16)  OutScaling=2^0  SaturateOnIntegerOverflow=on  OutDataTypeStr=Inherit: Same as input  ParamDataTypeStr=Inherit: Same as input
  Gain4 : Gain  Gain=5  ParameterDataType=sfix(16)  ParameterScaling=2^0  OutDataType=sfix(16)  OutScaling=2^0  SaturateOnIntegerOverflow=on  OutDataTypeStr=Inherit: Same as input  ParamDataTypeStr=Inherit: Same as input
  Gain5 : Gain  Gain=6  ParameterDataType=sfix(16)  ParameterScaling=2^0  OutDataType=sfix(16)  OutScaling=2^0  SaturateOnIntegerOverflow=on  OutDataTypeStr=Inherit: Same as input  ParamDataTypeStr=Inherit: Same as input
  Logical Operator{,1..5} (6 alike) : Logic
  Relational Operator{1,3,5,7,9,12} (6 alike) : RelationalOperator  Operator=<=  InputSameDT=on
  Relational Operator{2,4,6,8,10..11} (6 alike) : RelationalOperator  Operator=>  InputSameDT=on
  Saturation : Saturate  UpperLimit=6  LowerLimit=1
  Sum : Sum  Inputs=|++++++  OutDataType=sfix(16)  OutScaling=2^0  SaturateOnIntegerOverflow=on  InputSameDT=on  OutDataTypeStr=Inherit: Same as first input
  N : Outport  OutDataType=sfix(16)  OutScaling=2^0
  wires:
  Data Type Conversion5/1 -> Gain5/1
  Data Type Conversion4/1 -> Gain4/1
  Data Type Conversion3/1 -> Gain3/1
  Data Type Conversion2/1 -> Gain2/1
  Data Type Conversion1/1 -> Gain1/1
  Data Type Conversion/1 -> Gain/1
  Relational Operator2/1 -> Logical Operator/1
  Relational Operator1/1 -> Logical Operator/2
  Logical Operator/1 -> Data Type Conversion/1
  theta/1 -> Relational Operator2/1, Relational Operator1/1, Relational Operator4/1, Relational Operator3/1, Relational Operator6/1, Relational Operator5/1, Relational Operator8/1, Relational Operator7/1, Relational Operator10/1, Relational Operator9/1, Relational Operator11/1, Relational Operator12/1
  Constant/1 -> Relational Operator2/2
  Constant1/1 -> Relational Operator1/2
  Relational Operator4/1 -> Logical Operator1/1
  Relational Operator3/1 -> Logical Operator1/2
  Logical Operator1/1 -> Data Type Conversion1/1
  Constant2/1 -> Relational Operator4/2
  Constant3/1 -> Relational Operator3/2
  Relational Operator6/1 -> Logical Operator2/1
  Relational Operator5/1 -> Logical Operator2/2
  Logical Operator2/1 -> Data Type Conversion2/1
  Constant4/1 -> Relational Operator6/2
  Constant5/1 -> Relational Operator5/2
  Relational Operator8/1 -> Logical Operator3/1
  Relational Operator7/1 -> Logical Operator3/2
  Logical Operator3/1 -> Data Type Conversion3/1
  Constant6/1 -> Relational Operator8/2
  Constant7/1 -> Relational Operator7/2
  Relational Operator10/1 -> Logical Operator4/1
  Relational Operator9/1 -> Logical Operator4/2
  Logical Operator4/1 -> Data Type Conversion4/1
  Constant8/1 -> Relational Operator10/2
  Constant9/1 -> Relational Operator9/2
  Relational Operator11/1 -> Logical Operator5/1
  Relational Operator12/1 -> Logical Operator5/2
  Logical Operator5/1 -> Data Type Conversion5/1
  Constant10/1 -> Relational Operator11/2
  Constant11/1 -> Relational Operator12/2
  Gain/1 -> Sum/1
  Gain1/1 -> Sum/2
  Gain2/1 -> Sum/3
  Gain3/1 -> Sum/4
  Gain4/1 -> Sum/5
  Gain5/1 -> Sum/6
  Sum/1 -> Saturation/1
  Saturation/1 -> N/1

== system svpwm3level/svpwm/Vector status/I ==
  n : Inport  OutDataType=sfix(16)  OutScaling=2^0
  m : Inport  Port=2  OutDataType=sfix(16)  OutScaling=2^0
  1-1 : Subsystem
  1-2 : Subsystem
  1-3 : Subsystem
  1-4 : Subsystem
  1-5 : Subsystem
  1-6 : Subsystem
  Multiport Switch : MultiPortSwitch  Inputs=6  OutDataType=sfix(16)  OutScaling=2^0  InputSameDT=on
  State : Outport  OutDataType=sfix(16)  OutScaling=2^0
  wires:
  m/1 -> 1-1/1(m), 1-2/1(m), 1-3/1(m), 1-4/1(m), 1-5/1(m), 1-6/1(m)
  1-1/1(State) -> Multiport Switch/2
  1-2/1(State) -> Multiport Switch/3
  1-3/1(State) -> Multiport Switch/4
  1-4/1(State3) -> Multiport Switch/5
  1-5/1(State) -> Multiport Switch/6
  1-6/1(State5) -> Multiport Switch/7
  n/1 -> Multiport Switch/1
  Multiport Switch/1 -> State/1

== system svpwm3level/svpwm/Vector status/II ==
  n : Inport  OutDataType=sfix(16)  OutScaling=2^0
  m : Inport  Port=2  OutDataType=sfix(16)  OutScaling=2^0
  2-1 : Subsystem
  2-2 : Subsystem
  2-3 : Subsystem
  2-4 : Subsystem
  2-5 : Subsystem
  2-6 : Subsystem
  Multiport Switch1 : MultiPortSwitch  Inputs=6  OutDataType=sfix(16)  OutScaling=2^0  InputSameDT=on
  State : Outport  OutDataType=sfix(16)  OutScaling=2^0
  wires:
  m/1 -> 2-1/1(m), 2-2/1(m), 2-3/1(m), 2-4/1(m), 2-5/1(m), 2-6/1(m)
  2-1/1(State) -> Multiport Switch1/2
  2-2/1(State1) -> Multiport Switch1/3
  2-3/1(State2) -> Multiport Switch1/4
  2-4/1(State) -> Multiport Switch1/5
  2-5/1(State) -> Multiport Switch1/6
  2-6/1(State) -> Multiport Switch1/7
  n/1 -> Multiport Switch1/1
  Multiport Switch1/1 -> State/1

== system svpwm3level/svpwm/Vector status/III ==
  n : Inport  OutDataType=sfix(16)  OutScaling=2^0
  m : Inport  Port=2  OutDataType=sfix(16)  OutScaling=2^0
  3-1 : Subsystem
  3-2 : Subsystem
  3-3 : Subsystem
  3-4 : Subsystem
  3-5 : Subsystem
  3-6 : Subsystem
  Multiport Switch1 : MultiPortSwitch  Inputs=6  OutDataType=sfix(16)  OutScaling=2^0  InputSameDT=on
  State : Outport  OutDataType=sfix(16)  OutScaling=2^0
  wires:
  m/1 -> 3-1/1(m), 3-2/1(m), 3-3/1(m), 3-4/1(m), 3-5/1(m), 3-6/1(m)
  3-1/1(State) -> Multiport Switch1/2
  3-2/1(State) -> Multiport Switch1/3
  3-3/1(State2) -> Multiport Switch1/4
  3-4/1(State) -> Multiport Switch1/5
  3-5/1(State) -> Multiport Switch1/6
  3-6/1(State) -> Multiport Switch1/7
  n/1 -> Multiport Switch1/1
  Multiport Switch1/1 -> State/1

== system svpwm3level/svpwm/Vector status/IV ==
  n : Inport  OutDataType=sfix(16)  OutScaling=2^0
  m : Inport  Port=2  OutDataType=sfix(16)  OutScaling=2^0
  4-1 : Subsystem
  4-2 : Subsystem
  4-3 : Subsystem
  4-4 : Subsystem
  4-5 : Subsystem
  4-6 : Subsystem
  Multiport Switch1 : MultiPortSwitch  Inputs=6  OutDataType=sfix(16)  OutScaling=2^0  InputSameDT=on
  State : Outport  OutDataType=sfix(16)  OutScaling=2^0
  wires:
  m/1 -> 4-1/1(m), 4-2/1(m), 4-3/1(m), 4-4/1(m), 4-5/1(m), 4-6/1(m)
  4-1/1(State) -> Multiport Switch1/2
  4-2/1(State) -> Multiport Switch1/3
  4-3/1(State2) -> Multiport Switch1/4
  4-4/1(State) -> Multiport Switch1/5
  4-5/1(State4) -> Multiport Switch1/6
  4-6/1(State) -> Multiport Switch1/7
  n/1 -> Multiport Switch1/1
  Multiport Switch1/1 -> State/1

== system svpwm3level/svpwm/Vector status/V ==
  n : Inport  OutDataType=sfix(16)  OutScaling=2^0
  m : Inport  Port=2  OutDataType=sfix(16)  OutScaling=2^0
  5-1 : Subsystem
  5-2 : Subsystem
  5-3 : Subsystem
  5-4 : Subsystem
  5-5 : Subsystem
  5-6 : Subsystem
  Multiport Switch1 : MultiPortSwitch  Inputs=6  OutDataType=sfix(16)  OutScaling=2^0  InputSameDT=on
  State : Outport  OutDataType=sfix(16)  OutScaling=2^0
  wires:
  m/1 -> 5-1/1(m), 5-2/1(m), 5-3/1(m), 5-4/1(m), 5-5/1(m), 5-6/1(m)
  5-1/1(State) -> Multiport Switch1/2
  5-2/1(State1) -> Multiport Switch1/3
  5-3/1(State2) -> Multiport Switch1/4
  5-4/1(State3) -> Multiport Switch1/5
  5-5/1(State4) -> Multiport Switch1/6
  5-6/1(State) -> Multiport Switch1/7
  n/1 -> Multiport Switch1/1
  Multiport Switch1/1 -> State/1

== system svpwm3level/svpwm/Vector status/VI ==
  n : Inport  OutDataType=sfix(16)  OutScaling=2^0
  m : Inport  Port=2  OutDataType=sfix(16)  OutScaling=2^0
  6-1 : Subsystem
  6-2 : Subsystem
  6-3 : Subsystem
  6-4 : Subsystem
  6-5 : Subsystem
  6-6 : Subsystem
  Multiport Switch1 : MultiPortSwitch  Inputs=6  OutDataType=sfix(16)  OutScaling=2^0  InputSameDT=on
  State : Outport  OutDataType=sfix(16)  OutScaling=2^0
  wires:
  m/1 -> 6-1/1(m), 6-2/1(m), 6-3/1(m), 6-4/1(m), 6-5/1(m), 6-6/1(m)
  6-1/1(State) -> Multiport Switch1/2
  6-2/1(State) -> Multiport Switch1/3
  6-3/1(State2) -> Multiport Switch1/4
  6-4/1(State3) -> Multiport Switch1/5
  6-5/1(State4) -> Multiport Switch1/6
  6-6/1(State) -> Multiport Switch1/7
  n/1 -> Multiport Switch1/1
  Multiport Switch1/1 -> State/1

== system svpwm3level/svpwm/Subsystem1/Subsystem/n=1 ==
  Ta : Inport
  Tb : Inport  Port=2
  Tc : Inport  Port=3
  Ts : Inport  Port=4
  Add : Sum  Inputs=-+  OutDataType=fixdt(1, 16)  OutScaling=2^-10
  Mux : Mux  Inputs=3
  Scope1 : Scope  NumInputPorts=3
      settings: YMin=0.0001~-0.0013~2.71051e-020  YMax=0.0012~-0.001125~0.0011  SaveName=ScopeData13
  Tout : Outport
  wires:
  Ts/1 -> Add/2
  Mux/1 -> Tout/1
  Tb/1 -> Add/1
  Ta/1 -> Mux/1, Scope1/1
  Add/1 -> Mux/2, Scope1/2
  Tc/1 -> Mux/3, Scope1/3

== system svpwm3level/svpwm/Subsystem1/Subsystem/n=2 ==
  Ta : Inport
  Tb : Inport  Port=2
  Tc : Inport  Port=3
  Ts : Inport  Port=4
  Add : Sum  Inputs=-+  OutDataType=fixdt(1, 16)  OutScaling=2^-10
  Mux : Mux  Inputs=3
  Scope1 : Scope  NumInputPorts=3
      settings: YMin=0.0001~-0.0013~2.71051e-020  YMax=0.0012~-0.001125~0.0011  SaveName=ScopeData12
  Tout : Outport
  wires:
  Ts/1 -> Add/2
  Mux/1 -> Tout/1
  Tb/1 -> Add/1
  Add/1 -> Scope1/2, Mux/3
  Tc/1 -> Mux/1
  Ta/1 -> Mux/2

== system svpwm3level/svpwm/Subsystem1/Subsystem/n=3 ==
  Ta : Inport
  Tb : Inport  Port=2
  Tc : Inport  Port=3
  T : Inport  Port=4
  Add : Sum  Inputs=-+  OutDataType=fixdt(1, 16)  OutScaling=2^-10
  Add1 : Sum  Inputs=+-  OutDataType=fixdt(1, 16)  OutScaling=2^-10
  Gain : Gain  Gain=2  ParameterDataType=fixdt(1, 16)  ParameterScaling=2^0  OutDataType=fixdt(1, 16)  OutScaling=2^0
  Mux : Mux  Inputs=3
  Scope1 : Scope  NumInputPorts=3
      settings: YMin=-0.0003~2.71051e-020~-0.001  YMax=-0.000125~0.0011~0.0002  SaveName=ScopeData18
  Scope2 : Scope
      settings: YMin=0.00212  YMax=0.0023  SaveName=ScopeData23
  Tout : Outport
  wires:
  Mux/1 -> Tout/1
  T/1 -> Gain/1, Add1/2
  Gain/1 -> Add/2
  Add/1 -> Mux/1, Scope1/1
  Ta/1 -> Add1/1
  Add1/1 -> Mux/3, Scope1/3
  Tc/1 -> Mux/2, Scope1/2
  Tb/1 -> Add/1, Scope2/1

== system svpwm3level/svpwm/Subsystem1/Subsystem/n=4 ==
  Ta : Inport
  Tb : Inport  Port=2
  Tc : Inport  Port=3
  T : Inport  Port=4
  Add : Sum  Inputs=-+  OutDataType=fixdt(1, 16)  OutScaling=2^-10
  Add1 : Sum  Inputs=+-  OutDataType=fixdt(1, 16)  OutScaling=2^-10
  Add2 : Sum  Inputs=-+  OutDataType=fixdt(1, 16)  OutScaling=2^-10
  Mux : Mux  Inputs=3
  Scope1 : Scope  NumInputPorts=3
      settings: YMin=-0.0002~0.001125~-0.0002  YMax=0.001~0.0013~0.001  SaveName=ScopeData19
  Tout : Outport
  wires:
  Mux/1 -> Tout/1
  T/1 -> Add1/2, Add/2, Add2/2
  Add/1 -> Mux/1, Scope1/1
  Add1/1 -> Mux/2, Scope1/2
  Add2/1 -> Mux/3, Scope1/3
  Tb/1 -> Add1/1
  Tc/1 -> Add/1
  Ta/1 -> Add2/1

== system svpwm3level/svpwm/Subsystem1/Subsystem/n=5 ==
  Ta : Inport
  Tb : Inport  Port=2
  Tc : Inport  Port=3
  T : Inport  Port=4
  Add : Sum  Inputs=-+  OutDataType=fixdt(1, 16)  OutScaling=2^-10
  Add1 : Sum  Inputs=+-  OutDataType=fixdt(1, 16)  OutScaling=2^-10
  Add2 : Sum  Inputs=-+  OutDataType=fixdt(1, 16)  OutScaling=2^-10
  Mux : Mux  Inputs=3
  Scope1 : Scope  NumInputPorts=3
      settings: YMin=-0.0002~-0.0002~0.001125  YMax=0.001~0.001~0.0013  SaveName=ScopeData20
  Tout : Outport
  wires:
  Mux/1 -> Tout/1
  T/1 -> Add1/2, Add/2, Add2/2
  Ta/1 -> Add2/1
  Tc/1 -> Add/1
  Tb/1 -> Add1/1
  Add2/1 -> Mux/1, Scope1/1
  Add/1 -> Mux/2, Scope1/2
  Add1/1 -> Mux/3, Scope1/3

== system svpwm3level/svpwm/Subsystem1/Subsystem/n=6 ==
  Ta : Inport
  Tb : Inport  Port=2
  Tc : Inport  Port=3
  T : Inport  Port=4
  Add : Sum  Inputs=-+  OutDataType=fixdt(1, 16)  OutScaling=2^-10
  Add1 : Sum  Inputs=+-  OutDataType=fixdt(1, 16)  OutScaling=2^-10
  Gain : Gain  Gain=2  ParameterDataType=fixdt(1, 16)  ParameterScaling=2^0  OutDataType=fixdt(1, 16)  OutScaling=2^0
  Mux : Mux  Inputs=3
  Scope1 : Scope  NumInputPorts=3
      settings: YMin=0.0005~-0.002~-8.13152e-020  YMax=0.00075~-0.0005~0.0015  SaveName=ScopeData21
  Tout : Outport
  wires:
  Mux/1 -> Tout/1
  T/1 -> Gain/1, Add1/2
  Add/1 -> Mux/1, Scope1/1
  Tc/1 -> Add1/1
  Add1/1 -> Mux/2, Scope1/2
  Ta/1 -> Mux/3, Scope1/3
  Gain/1 -> Add/2
  Tb/1 -> Add/1

== system svpwm3level/svpwm/Vector status/I/1-1 ==
  m : Inport  OutDataType=sfix(16)  OutScaling=2^0
  Constant1 : Constant  Value="[0  0  0]"  OutDataType=sfix(16)  OutScaling=2^0
  Constant11 : Constant  Value=[0 0 -1]  OutDataType=sfix(16)  OutScaling=2^0
  Constant2 : Constant  Value=[0 -1 -1]  OutDataType=sfix(16)  OutScaling=2^0
  Constant3 : Constant  Value=[0 0 -1]  OutDataType=sfix(16)  OutScaling=2^0
  Constant4 : Constant  Value=[1 0 0]  OutDataType=sfix(16)  OutScaling=2^0
  Constant5 : Constant  Value=[1 0 0]  OutDataType=sfix(16)  OutScaling=2^0
  Constant6 : Constant  Value=[0 0 0]  OutDataType=sfix(16)  OutScaling=2^0
  Multiport Switch : MultiPortSwitch  Inputs=7  OutDataType=sfix(16)  OutScaling=2^0  InputSameDT=on
  State : Outport  OutDataType=sfix(16)  OutScaling=2^0
  wires:
  Constant5/1 -> Multiport Switch/2
  Constant6/1 -> Multiport Switch/3
  Constant11/1 -> Multiport Switch/4
  m/1 -> Multiport Switch/1
  Multiport Switch/1 -> State/1
  Constant2/1 -> Multiport Switch/5
  Constant3/1 -> Multiport Switch/6
  Constant1/1 -> Multiport Switch/7
  Constant4/1 -> Multiport Switch/8

== system svpwm3level/svpwm/Vector status/I/1-2 ==
  m : Inport  OutDataType=sfix(16)  OutScaling=2^0
  Constant10 : Constant  Value=[0 0 0]  OutDataType=sfix(16)  OutScaling=2^0
  Constant14 : Constant  Value=[1 1 0]  OutDataType=sfix(16)  OutScaling=2^0
  Constant5 : Constant  Value=[1 0 0]  OutDataType=sfix(16)  OutScaling=2^0
  Constant6 : Constant  Value=[0 0 0]  OutDataType=sfix(16)  OutScaling=2^0
  Constant7 : Constant  Value=[1 1 0]  OutDataType=sfix(16)  OutScaling=2^0
  Constant8 : Constant  Value=[1 0 0]  OutDataType=sfix(16)  OutScaling=2^0
  Constant9 : Constant  Value=[0 0 -1]  OutDataType=sfix(16)  OutScaling=2^0
  Multiport Switch1 : MultiPortSwitch  Inputs=7  OutDataType=sfix(16)  OutScaling=2^0  InputSameDT=on
  State : Outport  OutDataType=sfix(16)  OutScaling=2^0
  wires:
  Constant14/1 -> Multiport Switch1/8
  Constant5/1 -> Multiport Switch1/7
  Constant10/1 -> Multiport Switch1/6
  Constant9/1 -> Multiport Switch1/5
  Multiport Switch1/1 -> State/1
  m/1 -> Multiport Switch1/1
  Constant6/1 -> Multiport Switch1/4
  Constant8/1 -> Multiport Switch1/3
  Constant7/1 -> Multiport Switch1/2

== system svpwm3level/svpwm/Vector status/I/1-3 ==
  m : Inport  OutDataType=sfix(16)  OutScaling=2^0
  Constant1 : Constant  Value=[1 -1 -1]  OutDataType=sfix(16)  OutScaling=2^0
  Constant11 : Constant  Value=[1 0 0]  OutDataType=sfix(16)  OutScaling=2^0
  Constant12 : Constant  Value=[1 0 -1]  OutDataType=sfix(16)  OutScaling=2^0
  Constant13 : Constant  Value=[0 -1 -1]  OutDataType=sfix(16)  OutScaling=2^0
  Constant2 : Constant  Value=[1 0 0]  OutDataType=sfix(16)  OutScaling=2^0
  Constant3 : Constant  Value=[1 0 -1]  OutDataType=sfix(16)  OutScaling=2^0
  Constant4 : Constant  Value=[1 -1 -1]  OutDataType=sfix(16)  OutScaling=2^0
  Multiport Switch2 : MultiPortSwitch  Inputs=7  OutDataType=sfix(16)  OutScaling=2^0  InputSameDT=on
  State : Outport  OutDataType=sfix(16)  OutScaling=2^0
  wires:
  Constant2/1 -> Multiport Switch2/8
  Constant3/1 -> Multiport Switch2/7
  Constant1/1 -> Multiport Switch2/6
  Constant13/1 -> Multiport Switch2/5
  Multiport Switch2/1 -> State/1
  m/1 -> Multiport Switch2/1
  Constant4/1 -> Multiport Switch2/4
  Constant12/1 -> Multiport Switch2/3
  Constant11/1 -> Multiport Switch2/2

== system svpwm3level/svpwm/Vector status/I/1-4 ==
  m : Inport  OutDataType=sfix(16)  OutScaling=2^0
  Constant1 : Constant  Value=[0 0 -1]  OutDataType=sfix(16)  OutScaling=2^0
  Constant14 : Constant  Value=[0 0 -1]  OutDataType=sfix(16)  OutScaling=2^0
  Constant2 : Constant  Value=[1 0 -1]  OutDataType=sfix(16)  OutScaling=2^0
  Constant3 : Constant  Value=[1 0 0]  OutDataType=sfix(16)  OutScaling=2^0
  Constant6 : Constant  Value=[1 0 0]  OutDataType=sfix(16)  OutScaling=2^0
  Constant7 : Constant  Value=[1 0 -1]  OutDataType=sfix(16)  OutScaling=2^0
  Constant8 : Constant  Value=[0 -1 -1]  OutDataType=sfix(16)  OutScaling=2^0
  Multiport Switch1 : MultiPortSwitch  Inputs=7  OutDataType=sfix(16)  OutScaling=2^0  InputSameDT=on
  State3 : Outport  OutDataType=sfix(16)  OutScaling=2^0
  wires:
  Constant3/1 -> Multiport Switch1/8
  Constant2/1 -> Multiport Switch1/7
  Constant1/1 -> Multiport Switch1/6
  Constant8/1 -> Multiport Switch1/5
  Multiport Switch1/1 -> State3/1
  m/1 -> Multiport Switch1/1
  Constant14/1 -> Multiport Switch1/4
  Constant7/1 -> Multiport Switch1/3
  Constant6/1 -> Multiport Switch1/2

== system svpwm3level/svpwm/Vector status/I/1-5 ==
  m : Inport  OutDataType=sfix(16)  OutScaling=2^0
  Constant15 : Constant  Value="[1 0  0]"  OutDataType=sfix(16)  OutScaling=2^0
  Constant16 : Constant  Value=[1 0 -1]  OutDataType=sfix(16)  OutScaling=2^0
  Constant17 : Constant  Value=[1 0 -1]  OutDataType=sfix(16)  OutScaling=2^0
  Constant18 : Constant  Value=[1 1 0]  OutDataType=sfix(16)  OutScaling=2^0
  Constant19 : Constant  Value=[1 0 0]  OutDataType=sfix(16)  OutScaling=2^0
  Constant20 : Constant  Value=[0 0 -1]  OutDataType=sfix(16)  OutScaling=2^0
  Constant21 : Constant  Value=[1 1 0]  OutDataType=sfix(16)  OutScaling=2^0
  Multiport Switch3 : MultiPortSwitch  Inputs=7  OutDataType=sfix(16)  OutScaling=2^0  InputSameDT=on
  State : Outport  OutDataType=sfix(16)  OutScaling=2^0
  wires:
  Constant21/1 -> Multiport Switch3/8
  Constant15/1 -> Multiport Switch3/7
  Constant17/1 -> Multiport Switch3/6
  Constant20/1 -> Multiport Switch3/5
  Multiport Switch3/1 -> State/1
  m/1 -> Multiport Switch3/1
  Constant16/1 -> Multiport Switch3/4
  Constant19/1 -> Multiport Switch3/3
  Constant18/1 -> Multiport Switch3/2

== system svpwm3level/svpwm/Vector status/I/1-6 ==
  m : Inport  OutDataType=sfix(16)  OutScaling=2^0
  Constant22 : Constant  Value=[1 1 -1]  OutDataType=sfix(16)  OutScaling=2^0
  Constant23 : Constant  Value=[1 0 -1]  OutDataType=sfix(16)  OutScaling=2^0
  Constant24 : Constant  Value=[1 0 -1]  OutDataType=sfix(16)  OutScaling=2^0
  Constant25 : Constant  Value=[1 1 0]  OutDataType=sfix(16)  OutScaling=2^0
  Constant26 : Constant  Value=[1 1 -1]  OutDataType=sfix(16)  OutScaling=2^0
  Constant27 : Constant  Value=[0 0 -1]  OutDataType=sfix(16)  OutScaling=2^0
  Constant28 : Constant  Value=[1 1 0]  OutDataType=sfix(16)  OutScaling=2^0
  Multiport Switch4 : MultiPortSwitch  Inputs=7  OutDataType=sfix(16)  OutScaling=2^0  InputSameDT=on
  State5 : Outport  OutDataType=sfix(16)  OutScaling=2^0
  wires:
  Constant28/1 -> Multiport Switch4/8
  Constant22/1 -> Multiport Switch4/7
  Constant24/1 -> Multiport Switch4/6
  Constant27/1 -> Multiport Switch4/5
  Multiport Switch4/1 -> State5/1
  m/1 -> Multiport Switch4/1
  Constant23/1 -> Multiport Switch4/4
  Constant26/1 -> Multiport Switch4/3
  Constant25/1 -> Multiport Switch4/2
